simulink model "SimpleGeometrycModelOfGreenHouse"  (R2015a)
settings: Solver=ode45  StartTime=StartTimeSimulation  StopTime=EndTimeSimulation  MaxStep=0.1  RelTol=1e-3
libraries: simulink x3
settings Model: SimulationMode=accelerator  CovSFcnEnable=off  Creator=Oleg_2  LastModifiedBy=Oleg_2
settings DataIOCC: LimitDataPoints=off  SaveOutput=off  SignalLogging=off  DSMLogging=off  SaveTime=off
settings DebuggingCC: UnderspecifiedInitializationDetection=Classic  MergeDetectMultiDrivingBlocksExec=none

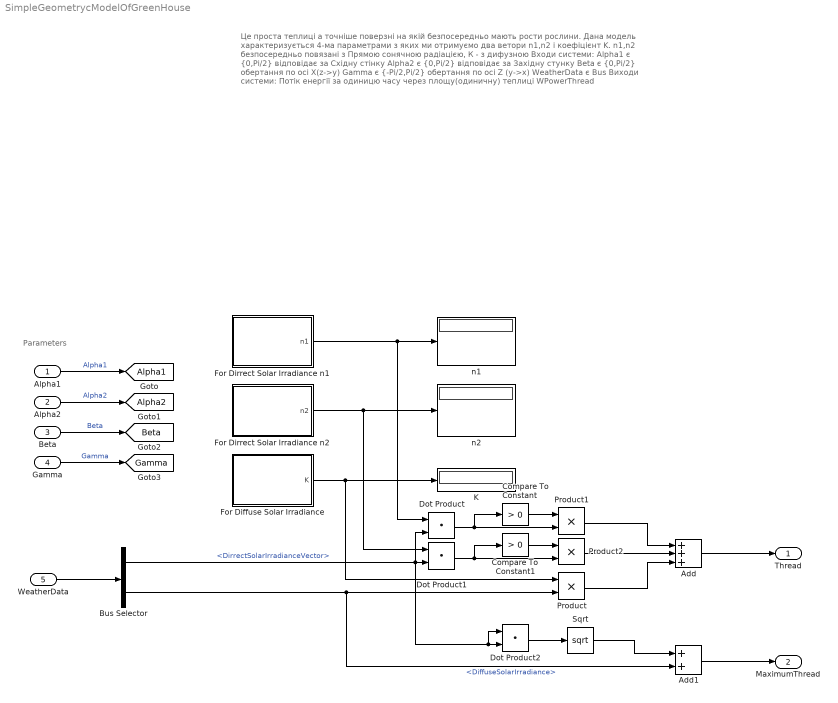
== system SimpleGeometrycModelOfGreenHouse ==
  note: Parameters
  note: Це проста теплиці а точніше поверзні на якій безпосередньо
      | мають рости рослини. Дана модель характеризується 4-ма параметрами
      | з яких ми отримуємо два ветори n1,n2 і коефіцієнт K.
      |
      | n1,n2 безпосередньо повязані з Прямою сонячною радіацією,
      | К - з дифузною
      |
      | Входи системи:
      | Alpha1 є {0,Pi/2} відповідає за Східну стінку
      | Alpha2 є {0,Pi/2} відповідає за Західну стунку
      | Beta є {0,Pi/2} обертання по осі Х(z->y)
      | Gamma є {-Pi/2,Pi/2} обертання по осі Z (y->x)
      |
      | WeatherData є Bus
      | Виходи системи:
      | Потік енергії за одиницю часу через площу(одиничну) теплиці
      | WPowerThread
  Alpha1 : Inport  OutDataTypeStr=double  PortDimensions=1  SampleTime=0
  Alpha2 : Inport  Port=2  OutDataTypeStr=double  PortDimensions=1  SampleTime=0
  Beta : Inport  Port=3  OutDataTypeStr=double  PortDimensions=1  SampleTime=0
  Gamma : Inport  Port=4  OutDataTypeStr=double  PortDimensions=1  SampleTime=0
  WeatherData : Inport  Port=5  OutDataTypeStr=Bus: WeatherData  SampleTime=0  Interpolate=off
  Add : Sum  Inputs=+++
  Add1 : Sum
  Bus Selector : BusSelector  OutputSignals=DirrectSolarIrradianceVector,DiffuseSolarIrradiance
  Compare To Constant : simulink/Logic and Bit Operations/Compare To Constant  relop=>  const=0  OutDataTypeStr=boolean
  Compare To Constant1 : simulink/Logic and Bit Operations/Compare To Constant  relop=>  const=0  OutDataTypeStr=boolean
  Dot Product : DotProduct  InputSameDT=on  OutDataTypeStr=Inherit: Inherit via internal rule
  Dot Product1 : DotProduct  InputSameDT=on  OutDataTypeStr=Inherit: Inherit via internal rule
  Dot Product2 : DotProduct  InputSameDT=on  OutDataTypeStr=Inherit: Inherit via internal rule
  For Diffuse Solar Irradiance : Subsystem
  For Dirrect Solar Irradiance n1 : Subsystem
  For Dirrect Solar Irradiance n2 : Subsystem
  K : Display
  Product : Product
  Product1 : Product
  Product2 : Product
  Sqrt : Sqrt  SaturateOnIntegerOverflow=on
  n1 : Display
  n2 : Display
  Thread : Outport
  MaximumThread : Outport  Port=2
  tag scope: Alpha1=global, Alpha2=global, Beta=global, Gamma=global
  wires:
  WeatherData/1 -> Bus Selector/1
  Alpha1/1 -> [Alpha1]  "Alpha1"
  Alpha2/1 -> [Alpha2]  "Alpha2"
  Beta/1 -> [Beta]  "Beta"
  Gamma/1 -> [Gamma]  "Gamma"
  Product/1 -> Add/3
  Bus Selector/2 -> Product/2, Add1/2  "<DiffuseSolarIrradiance>"
  For Diffuse Solar Irradiance/1(K) -> Product/1, K/1
  Bus Selector/1 -> Dot Product2/1, Dot Product2/2, Dot Product1/2, Dot Product/2  "<DirrectSolarIrradianceVector>"
  For Dirrect Solar Irradiance n2/1(n2) -> n2/1, Dot Product1/1
  Dot Product/1 -> Product1/2, Compare To Constant/1
  Compare To Constant/1 -> Product1/1
  Dot Product1/1 -> Product2/2, Compare To Constant1/1
  Compare To Constant1/1 -> Product2/1
  For Dirrect Solar Irradiance n1/1(n1) -> Dot Product/1, n1/1
  Product1/1 -> Add/1
  Product2/1 -> Add/2
  Add/1 -> Thread/1
  Dot Product2/1 -> Sqrt/1
  Add1/1 -> MaximumThread/1
  Sqrt/1 -> Add1/1

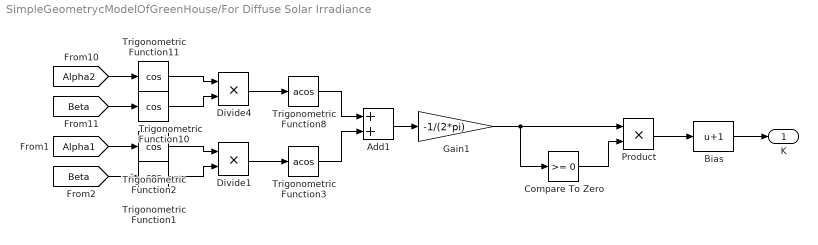
== system SimpleGeometrycModelOfGreenHouse/For Diffuse Solar Irradiance ==
  Add1 : Sum
  Bias : Bias  Bias=1
  Compare To Zero : simulink/Logic and Bit Operations/Compare To Zero  relop=>=  OutDataTypeStr=boolean
  Divide1 : Product  Inputs=**
  Divide4 : Product  Inputs=**
  Gain1 : Gain  Gain=-1/(2*pi)
  Product : Product
  Trigonometric Function{1..2,10..11} (4 alike) : Trigonometry  Operator=cos  OutputSignalType=real
  Trigonometric Function3 : Trigonometry  Operator=acos  OutputSignalType=real
  Trigonometric Function8 : Trigonometry  Operator=acos  OutputSignalType=real
  K : Outport
  wires:
  Bias/1 -> K/1
  Trigonometric Function8/1 -> Add1/1
  Gain1/1 -> Compare To Zero/1, Product/1
  Trigonometric Function3/1 -> Add1/2
  Add1/1 -> Gain1/1
  [Beta] -> Trigonometric Function10/1
  [Alpha2] -> Trigonometric Function11/1
  Trigonometric Function11/1 -> Divide4/1
  Trigonometric Function10/1 -> Divide4/2
  [Beta] -> Trigonometric Function1/1
  [Alpha1] -> Trigonometric Function2/1
  Trigonometric Function1/1 -> Divide1/2
  Divide1/1 -> Trigonometric Function3/1
  Trigonometric Function2/1 -> Divide1/1
  Divide4/1 -> Trigonometric Function8/1
  Compare To Zero/1 -> Product/2
  Product/1 -> Bias/1

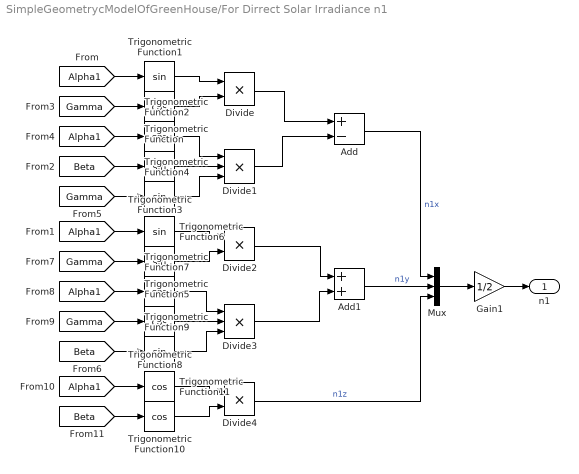
== system SimpleGeometrycModelOfGreenHouse/For Dirrect Solar Irradiance n1 ==
  Add : Sum  Inputs=+-
  Add1 : Sum
  Divide : Product  Inputs=**
  Divide1 : Product  Inputs=***
  Divide2 : Product  Inputs=**
  Divide3 : Product  Inputs=***
  Divide4 : Product  Inputs=**
  Gain1 : Gain  Gain=1/2
  Mux : Mux  Inputs=3
  Trigonometric Function{,2,7..8,10..11} (6 alike) : Trigonometry  Operator=cos  OutputSignalType=real
  Trigonometric Function{1,3..6,9} (6 alike) : Trigonometry  OutputSignalType=real
  n1 : Outport  OutDataTypeStr=double  PortDimensions=3
  wires:
  Trigonometric Function4/1 -> Divide1/3
  Divide3/1 -> Add1/2
  Trigonometric Function3/1 -> Divide1/2
  [Gamma] -> Trigonometric Function4/1
  Divide1/1 -> Add/2
  Trigonometric Function/1 -> Divide/2
  [Alpha1] -> Trigonometric Function1/1
  [Gamma] -> Trigonometric Function/1
  Divide/1 -> Add/1
  Trigonometric Function2/1 -> Divide1/1
  Trigonometric Function1/1 -> Divide/1
  Mux/1 -> Gain1/1
  Divide4/1 -> Mux/3  "n1z"
  Trigonometric Function11/1 -> Divide4/1
  Trigonometric Function10/1 -> Divide4/2
  [Beta] -> Trigonometric Function10/1
  [Alpha1] -> Trigonometric Function11/1
  Add1/1 -> Mux/2  "n1y"
  [Beta] -> Trigonometric Function3/1
  Add/1 -> Mux/1  "n1x"
  [Alpha1] -> Trigonometric Function2/1
  Trigonometric Function6/1 -> Divide2/1
  Divide2/1 -> Add1/1
  [Gamma] -> Trigonometric Function8/1
  [Beta] -> Trigonometric Function9/1
  Trigonometric Function5/1 -> Divide2/2
  Trigonometric Function9/1 -> Divide3/3
  [Gamma] -> Trigonometric Function5/1
  Trigonometric Function8/1 -> Divide3/2
  [Alpha1] -> Trigonometric Function7/1
  [Alpha1] -> Trigonometric Function6/1
  Trigonometric Function7/1 -> Divide3/1
  Gain1/1 -> n1/1

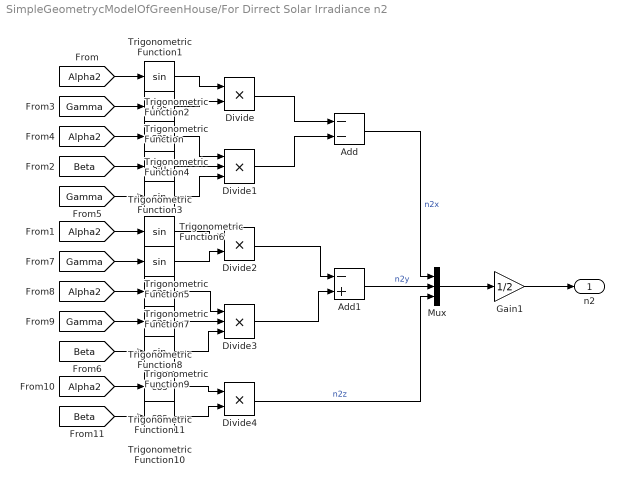
== system SimpleGeometrycModelOfGreenHouse/For Dirrect Solar Irradiance n2 ==
  Add : Sum  Inputs=--
  Add1 : Sum  Inputs=-+
  Divide : Product  Inputs=**
  Divide1 : Product  Inputs=***
  Divide2 : Product  Inputs=**
  Divide3 : Product  Inputs=***
  Divide4 : Product  Inputs=**
  Gain1 : Gain  Gain=1/2
  Mux : Mux  Inputs=3
  Trigonometric Function{,2,7..8,10..11} (6 alike) : Trigonometry  Operator=cos  OutputSignalType=real
  Trigonometric Function{1,3..6,9} (6 alike) : Trigonometry  OutputSignalType=real
  n2 : Outport  OutDataTypeStr=double  PortDimensions=3
  wires:
  Trigonometric Function4/1 -> Divide1/3
  Divide3/1 -> Add1/2
  Trigonometric Function3/1 -> Divide1/2
  [Gamma] -> Trigonometric Function4/1
  Divide1/1 -> Add/2
  Trigonometric Function/1 -> Divide/2
  [Alpha2] -> Trigonometric Function1/1
  [Gamma] -> Trigonometric Function/1
  Divide/1 -> Add/1
  Trigonometric Function2/1 -> Divide1/1
  Trigonometric Function1/1 -> Divide/1
  Mux/1 -> Gain1/1
  Divide4/1 -> Mux/3  "n2z"
  Trigonometric Function11/1 -> Divide4/1
  Trigonometric Function10/1 -> Divide4/2
  [Beta] -> Trigonometric Function10/1
  [Alpha2] -> Trigonometric Function11/1
  Add1/1 -> Mux/2  "n2y"
  [Beta] -> Trigonometric Function3/1
  Add/1 -> Mux/1  "n2x"
  [Alpha2] -> Trigonometric Function2/1
  Trigonometric Function6/1 -> Divide2/1
  Divide2/1 -> Add1/1
  [Gamma] -> Trigonometric Function8/1
  [Beta] -> Trigonometric Function9/1
  Trigonometric Function5/1 -> Divide2/2
  Trigonometric Function9/1 -> Divide3/3
  [Gamma] -> Trigonometric Function5/1
  Trigonometric Function8/1 -> Divide3/2
  [Alpha2] -> Trigonometric Function7/1
  [Alpha2] -> Trigonometric Function6/1
  Trigonometric Function7/1 -> Divide3/1
  Gain1/1 -> n2/1
